simulink model "step6"  (Simulink 8.1)
settings: Solver=ode45  StartTime=0.0  StopTime=20  RelTol=1e-3
values from neighbouring files (symbols this model uses):
  A = [0.8 0.3; 0 -0.6]    [setup.m]
  P = dlyap(A',Q)    [setup.m]
  x0 = [1;-0.5]    [setup.m]
libraries: simulink x6
settings Model: Creator=aeagr  LastModifiedBy=aeagr
settings DebuggingCC: FcnCallInpInsideContextMsg=EnableAllAsWarning
settings GRTTargetCC: CombineOutputUpdateFcns=on  GRTInterface=off

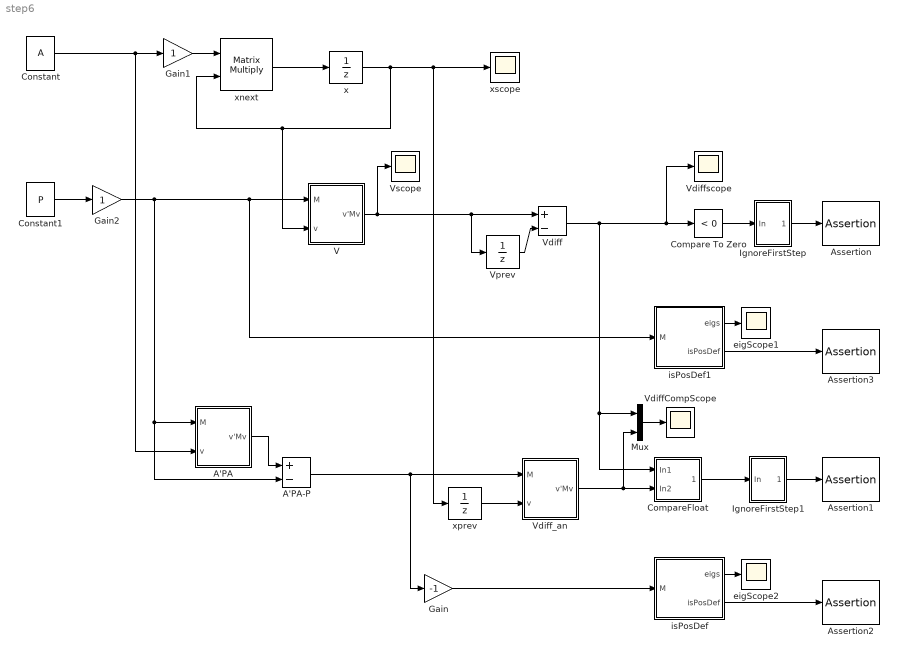
== system step6 ==
  A'PA : Subsystem
  A'PA-P : Sum  Inputs=+-
  Assertion : Assertion  Enabled=off
  Assertion1 : Assertion
  Assertion2 : Assertion
  Assertion3 : Assertion
  Compare To Zero : simulink/Logic and Bit Operations/Compare To Zero  relop=<  OutDataTypeStr=boolean
  CompareFloat : Subsystem
  Constant : Constant  Value=A
  Constant1 : Constant  Value=P
  Gain : Gain  Gain=-1
  Gain1 : Gain
  Gain2 : Gain
  IgnoreFirstStep : Subsystem
  IgnoreFirstStep1 : Subsystem
  Mux : Mux  Inputs=2
  V : Subsystem
  Vdiff : Sum  Inputs=+-
  VdiffCompScope : Scope
      settings: SaveName=ScopeData3
  Vdiff_an : Subsystem
  Vdiffscope : Scope
  Vprev : UnitDelay
  Vscope : Scope
      settings: SaveName=ScopeData2
  eigScope1 : Scope
      settings: SaveName=ScopeData5
  eigScope2 : Scope
      settings: SaveName=ScopeData4
  isPosDef : Subsystem
  isPosDef1 : Subsystem
  x : UnitDelay  InitialCondition=x0
  xnext : Product  Multiplication=Matrix(*)  RndMeth=Zero
  xprev : UnitDelay  InitialCondition=x0
  xscope : Scope
  wires:
  Constant/1 -> Gain1/1, A'PA/2(v)
  xnext/1 -> x/1
  x/1 -> xnext/2, V/2(v), xprev/1, xscope/1
  V/1(v'Mv) -> Vscope/1, Vprev/1, Vdiff/1
  Vprev/1 -> Vdiff/2
  Vdiff/1 -> Compare To Zero/1, Vdiffscope/1, CompareFloat/1(In1), Mux/1
  IgnoreFirstStep/1(Out) -> Assertion/1
  Compare To Zero/1 -> IgnoreFirstStep/1(In)
  A'PA/1(v'Mv) -> A'PA-P/1
  Vdiff_an/1(v'Mv) -> CompareFloat/2(In2), Mux/2
  xprev/1 -> Vdiff_an/2(v)
  Mux/1 -> VdiffCompScope/1
  CompareFloat/1(Out1) -> IgnoreFirstStep1/1(In)
  IgnoreFirstStep1/1(Out) -> Assertion1/1
  isPosDef/2(isPosDef) -> Assertion2/1
  Gain/1 -> isPosDef/1(M)
  isPosDef/1(eigs) -> eigScope2/1
  isPosDef1/2(isPosDef) -> Assertion3/1
  isPosDef1/1(eigs) -> eigScope1/1
  A'PA-P/1 -> Gain/1, Vdiff_an/1(M)
  Constant1/1 -> Gain2/1
  Gain1/1 -> xnext/1
  Gain2/1 -> A'PA/1(M), A'PA-P/2, V/1(M), isPosDef1/1(M)

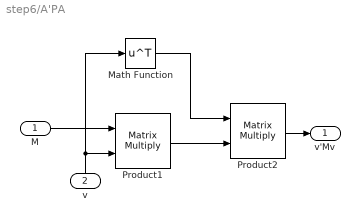
== system step6/A'PA ==
  M : Inport
  v : Inport  Port=2
  Math Function : Math  Operator=transpose  SaturateOnIntegerOverflow=on
  Product1 : Product  Multiplication=Matrix(*)  RndMeth=Zero
  Product2 : Product  Multiplication=Matrix(*)  RndMeth=Zero
  v'Mv : Outport
  wires:
  Product2/1 -> v'Mv/1
  M/1 -> Product1/1
  v/1 -> Product1/2, Math Function/1
  Math Function/1 -> Product2/1
  Product1/1 -> Product2/2

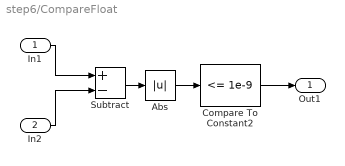
== system step6/CompareFloat ==
  In1 : Inport
  In2 : Inport  Port=2
  Abs : Abs
  Compare To Constant2 : simulink/Logic and Bit Operations/Compare To Constant  relop=<=  const=1e-9  OutDataTypeStr=boolean
  Subtract : Sum  Inputs=+-
  Out1 : Outport
  wires:
  Subtract/1 -> Abs/1
  Abs/1 -> Compare To Constant2/1
  In1/1 -> Subtract/1
  Compare To Constant2/1 -> Out1/1
  In2/1 -> Subtract/2

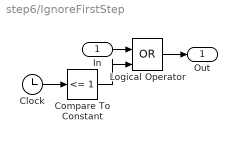
== system step6/IgnoreFirstStep ==
  In : Inport
  Clock : Clock
  Compare To Constant : simulink/Logic and Bit Operations/Compare To Constant  relop=<=  const=1  OutDataTypeStr=boolean
  Logical Operator : Logic  Operator=OR  IconShape=distinctive  AllPortsSameDT=off  OutDataTypeStr=boolean
  Out : Outport
  wires:
  Clock/1 -> Compare To Constant/1
  Compare To Constant/1 -> Logical Operator/2
  In/1 -> Logical Operator/1
  Logical Operator/1 -> Out/1

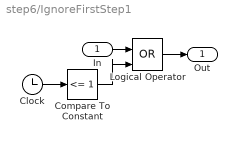
== system step6/IgnoreFirstStep1 ==
  In : Inport
  Clock : Clock
  Compare To Constant : simulink/Logic and Bit Operations/Compare To Constant  relop=<=  const=1  OutDataTypeStr=boolean
  Logical Operator : Logic  Operator=OR  IconShape=distinctive  AllPortsSameDT=off  OutDataTypeStr=boolean
  Out : Outport
  wires:
  Logical Operator/1 -> Out/1
  In/1 -> Logical Operator/1
  Compare To Constant/1 -> Logical Operator/2
  Clock/1 -> Compare To Constant/1

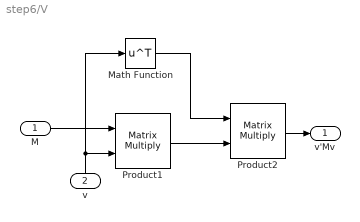
== system step6/V ==
  M : Inport
  v : Inport  Port=2
  Math Function : Math  Operator=transpose  SaturateOnIntegerOverflow=on
  Product1 : Product  Multiplication=Matrix(*)  RndMeth=Zero
  Product2 : Product  Multiplication=Matrix(*)  RndMeth=Zero
  v'Mv : Outport
  wires:
  Product1/1 -> Product2/2
  Math Function/1 -> Product2/1
  v/1 -> Math Function/1, Product1/2
  M/1 -> Product1/1
  Product2/1 -> v'Mv/1

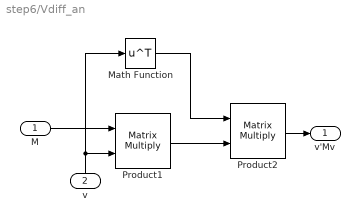
== system step6/Vdiff_an ==
  M : Inport
  v : Inport  Port=2
  Math Function : Math  Operator=transpose  SaturateOnIntegerOverflow=on
  Product1 : Product  Multiplication=Matrix(*)  RndMeth=Zero
  Product2 : Product  Multiplication=Matrix(*)  RndMeth=Zero
  v'Mv : Outport
  wires:
  Product2/1 -> v'Mv/1
  M/1 -> Product1/1
  v/1 -> Product1/2, Math Function/1
  Math Function/1 -> Product2/1
  Product1/1 -> Product2/2

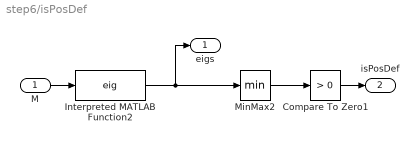
== system step6/isPosDef ==
  M : Inport
  Compare To Zero1 : simulink/Logic and Bit Operations/Compare To Zero  relop=>  OutDataTypeStr=boolean
  Interpreted MATLAB Function2 : MATLABFcn  MATLABFcn=eig
  MinMax2 : MinMax
  eigs : Outport
  isPosDef : Outport  Port=2
  wires:
  MinMax2/1 -> Compare To Zero1/1
  Interpreted MATLAB Function2/1 -> MinMax2/1, eigs/1
  Compare To Zero1/1 -> isPosDef/1
  M/1 -> Interpreted MATLAB Function2/1

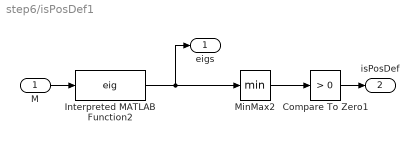
== system step6/isPosDef1 ==
  M : Inport
  Compare To Zero1 : simulink/Logic and Bit Operations/Compare To Zero  relop=>  OutDataTypeStr=boolean
  Interpreted MATLAB Function2 : MATLABFcn  MATLABFcn=eig
  MinMax2 : MinMax
  eigs : Outport
  isPosDef : Outport  Port=2
  wires:
  M/1 -> Interpreted MATLAB Function2/1
  Compare To Zero1/1 -> isPosDef/1
  Interpreted MATLAB Function2/1 -> eigs/1, MinMax2/1
  MinMax2/1 -> Compare To Zero1/1
